simulink model "helicopter_EKF"  (R2021b)
settings: Solver=ode45  StartTime=0.0  StopTime=T  RelTol=1e-3
InitFcn:
  | hwinit
values from neighbouring files (symbols this model uses):
  C = [1, 0, 0; 0, 0, 1]    [controller_LQR.m]    (also in controller_check_EKF.m; polish_MPC.m)
  h = 0.01    [controller_LQR.m]    (also in controller_check_EKF.m; observer_check_EKF.m; polish_MPC.m; validation.m)
  K = place(A_lin, B_lin, p_new)    [controller_check_EKF.m]
  u_start = alpha_to_u(alpha_ref)    [controller_LQR.m]
  x_ref = [alpha_ref; alpha_dot_ref; omega_ref]/0.9    [controller_LQR.m]    (also in controller_check_EKF.m = [alpha_ref; alpha_dot_ref; omega_ref]; polish_MPC.m = [alpha_ref; alpha_dot_ref ; omega_ref])
undefined symbols (not defined in the file or in its folder): A_lin, adingain, adinoffs, B_lin, HeliMexHandle
libraries: simulink x1, sharedTrackingLibrary x1, eeGeneralControl x1, dspstat3 x1
settings Model: Creator=fkzhang  LastModifiedBy=lcaric
settings SolverCC: AlgebraicLoopSolver=TrustRegion
settings DataIOCC: LimitDataPoints=on  SaveFormat=Array  ReturnWorkspaceOutputs=off
settings OptimizationCC: BlockReduction=off  BooleanDataType=off  LifeSpan=inf
settings DebuggingCC: SaveWithParameterizedLinksMsg=none  UnderspecifiedInitializationDetection=Classic  MergeDetectMultiDrivingBlocksExec=none  SignalResolutionControl=TryResolveAllWithWarning  AllowSymbolicDim=off  SFUnexpectedBacktrackingDiag=warning  SFNoUnconditionalDefaultTransitionDiag=warning  SFExecutionAtInitializationDiag=none  SFMachineParentedDataDiag=warning  ArithmeticOperatorsInVariantConditions=warning
settings HardwareCC: ProdBitPerPointer=32  ProdBitPerSizeT=32  ProdBitPerPtrDiffT=32  ProdLargestAtomicFloat=None  ProdIntDivRoundTo=Undefined  ProdEndianess=Unspecified  ProdWordSize=32  ProdHWDeviceType=32-bit Generic  TargetUnknown=on
settings ModelReferenceCC: PropagateSignalLabelsOutOfModel=off
settings SFSimCC: SimUseLocalCustomCode=off  CustomCodeUndefinedFunction=UseInterfaceOnly
settings RTWCC: RTWUseLocalCustomCode=off
settings CodeAppCC: StateflowObjectComments=on
settings GRTTargetCC: TargetLangStandard=C89/C90 (ANSI)
settings ConfigComp: CovMetricSettings=dw  CovSaveCumulativeToWorkspaceVar=on  CovSaveSingleToWorkspaceVar=on  CovExternalEMLEnable=off  CovSFcnEnable=off

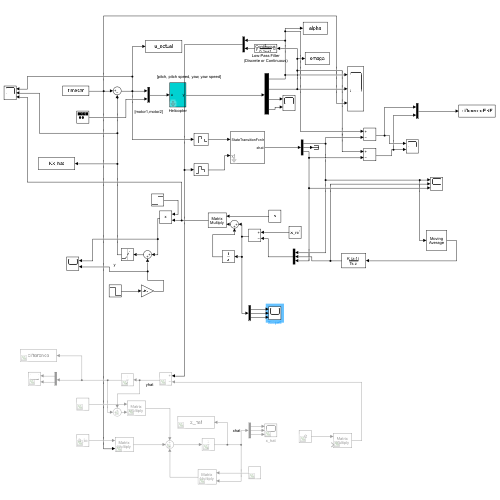
[thumbnail: Simulink's stored preview of the top-level diagram]
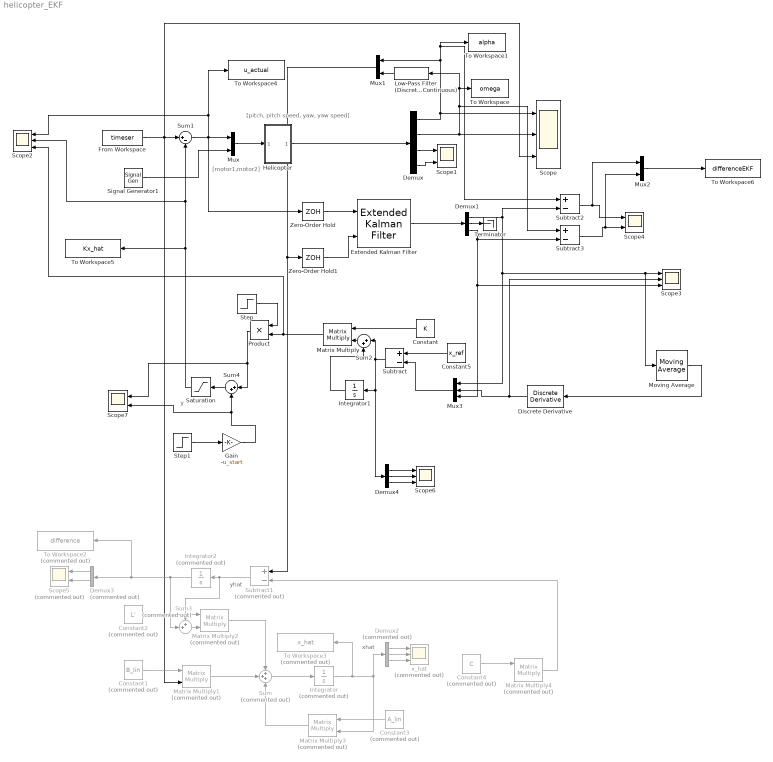
== system helicopter_EKF ==
  note: yhat
  note: y
  note: xhat
  note: [pitch, pitch speed, yaw, yaw speed]
  note: [motor1,motor2]
  Constant : Constant  Value=K  VectorParams1D=off
  Constant1 : Constant  Commented=on  Value=B_lin  VectorParams1D=off
  Constant2 : Constant  Commented=on  Value=L'
  Constant3 : Constant  Commented=on  Value=A_lin
  Constant4 : Constant  Commented=on  Value=C
  Constant5 : Constant  Value=x_ref
  Demux : Demux
  Demux1 : Demux  Outputs=3
  Demux2 : Demux  Commented=on  Outputs=3
  Demux3 : Demux  Commented=on  Outputs=2
  Demux4 : Demux  Outputs=3
  Discrete Derivative : simulink/Discrete/Discrete Derivative  gainval=1.0  ICPrevScaledInput=0.0  OutMin=[]  OutMax=[]  OutDataType=fixdt(1, 16)  OutScaling=2^-10  DoSatur=off
  Extended Kalman Filter : sharedTrackingLibrary/Extended Kalman Filter  StateTransitionFcn=nonlin_evolution  HasStateTransitionJacobianFcn=off  StateTransitionJacobianFcn=nonlin_jacobian  HasAdditiveProcessNoise=Additive  ProcessNoise=Q  HasTimeVaryingProcessNoise=off  HasStateTransitionFcnExtraArgument=1  InitialState=[0; 0; 0]  InitialStateCovariance=Q  MeasurementFcn1=nonlin_measurement_all  HasMeasurementJacobianFcn1=off  HasMeasurementEnablePort1=off  HasAdditiveMeasurementNoise1=Additive  MeasurementNoise1=R  HasTimeVaryingMeasurementNoise1=off  HasMeasurementFcnExtraArgument1=0  MeasurementFcn2=nonlin_measurement_omega  HasMeasurementJacobianFcn2=off  HasMeasurementEnablePort2=off  HasAdditiveMeasurementNoise2=Additive  MeasurementNoise2=10  HasTimeVaryingMeasurementNoise2=off  HasMeasurementFcnExtraArgument2=0  MeasurementFcn3=myMeasurementFcn  HasMeasurementJacobianFcn3=off  HasMeasurementEnablePort3=off  HasAdditiveMeasurementNoise3=Additive  MeasurementNoise3=1  HasTimeVaryingMeasurementNoise3=off  HasMeasurementFcnExtraArgument3=0  MeasurementFcn4=myMeasurementFcn  HasMeasurementJacobianFcn4=off  HasMeasurementEnablePort4=off  HasAdditiveMeasurementNoise4=Additive  MeasurementNoise4=1  HasTimeVaryingMeasurementNoise4=off  HasMeasurementFcnExtraArgument4=0  MeasurementFcn5=myMeasurementFcn  HasMeasurementJacobianFcn5=off  HasMeasurementEnablePort5=off  HasAdditiveMeasurementNoise5=Additive  MeasurementNoise5=1  HasTimeVaryingMeasurementNoise5=off  HasMeasurementFcnExtraArgument5=0  EnableMultirate=off  StateTransitionFcnSampleTime=1  MeasurementFcn1SampleTime=1  MeasurementFcn2SampleTime=1  MeasurementFcn3SampleTime=1  MeasurementFcn4SampleTime=1  MeasurementFcn5SampleTime=1  UseCurrentEstimator=on  OutputStateCovariance=off  DataType=double  SampleTime=0.02  NumberOfMeasurements=1
      settings: SourceProductBaseCode=AE,PW,CT,DR,TF,ID,LP,NV,AR,RO,RR,UV,VE
  From Workspace : FromWorkspace  VariableName=timeser
  Gain : Gain  Gain=-u_start
  Helicopter : Subsystem  mask{Ts=h}
      mask prompts: Ts "sampletime"
      mask init:
      | sf_heli_init
      mask Display:
      | port_label('input',1,'u');
      | port_label('output',1,'y');
  Integrator : Integrator  Commented=on
  Integrator1 : Integrator
  Integrator2 : Integrator  Commented=on
  Low-Pass Filter (Discrete or Continuous) : eeGeneralControl/Low-Pass Filter (Discrete or Continuous)  K=1  T=0.1  B=inf  A=-inf  init_option=Inherited from block input  x0=0  Ts=0
  Matrix Multiply : Product  Multiplication=Matrix(*)
  Matrix Multiply{1..4} (4 alike) : Product  Commented=on  Multiplication=Matrix(*)
  Moving Average : dspstat3/Moving Average  Method=Sliding window  ForgettingFactorPort=off  SpecifyWindowLength=on  WindowLength=5  ForgettingFactor=0.9  SimulateUsing=Code generation
  Mux : Mux  Inputs=2
  Mux1 : Mux  Inputs=2
  Mux2 : Mux  Inputs=2
  Mux3 : Mux  Inputs=3
  Product : Product
  Saturation : Saturate  UpperLimit=1  LowerLimit=-1
  Scope{,2..3,6} (4 alike) : Scope  NumInputPorts=3
  Scope1 : Scope  NumInputPorts=2
  Scope4 : Scope  NumInputPorts=2
  Scope5 : Scope  Commented=on  NumInputPorts=2
  Scope7 : Scope  NumInputPorts=2
  Signal Generator1 : SignalGenerator  WaveForm=square  Amplitude=0  Frequency=1/20
  Step : Step  SampleTime=0
  Step1 : Step  Before=1  After=0  SampleTime=0
  Subtract : Sum  Inputs=+-
  Subtract1 : Sum  Commented=on  Inputs=+-
  Subtract2 : Sum  Inputs=+-
  Subtract3 : Sum  Inputs=+-
  Sum : Sum  Commented=on  Inputs=+++
  Sum1 : Sum  Inputs=|+-
  Sum2 : Sum  Inputs=|++
  Sum3 : Sum  Commented=on  Inputs=++|
  Sum4 : Sum  Inputs=|++
  Terminator : Terminator
  To Workspace : ToWorkspace  VariableName=omega  SaveFormat=Timeseries  SampleTime=-1
  To Workspace1 : ToWorkspace  VariableName=alpha  SaveFormat=Timeseries  SampleTime=-1
  To Workspace2 : ToWorkspace  Commented=on  VariableName=difference  SaveFormat=Timeseries  SampleTime=-1
  To Workspace3 : ToWorkspace  Commented=on  VariableName=x_hat  SaveFormat=Timeseries  SampleTime=-1
  To Workspace4 : ToWorkspace  VariableName=u_actual  SaveFormat=Timeseries  SampleTime=-1
  To Workspace5 : ToWorkspace  VariableName=Kx_hat  SaveFormat=Timeseries  SampleTime=-1
  To Workspace6 : ToWorkspace  VariableName=differenceEKF  SaveFormat=Timeseries  SampleTime=-1
  Zero-Order Hold : ZeroOrderHold  SampleTime=0.02
  Zero-Order Hold1 : ZeroOrderHold  SampleTime=0.02
  x_hat : Scope  Commented=on  NumInputPorts=3
  wires:
  Mux/1 -> Helicopter/1(In1)
  Signal Generator1/1 -> Mux/2
  Demux/2 -> Low-Pass Filter (Discrete or Continuous)/1, To Workspace/1, Subtract3/1, Scope/2
  Demux/3 -> Scope1/1
  Demux/4 -> Scope1/2
  From Workspace/1 -> Sum1/1, Matrix Multiply1/2, Scope/3
  Demux/1 -> Subtract2/1, To Workspace1/1, Mux1/1, Scope/1
  Mux1/1 -> Subtract1/1, Zero-Order Hold1/1
  Helicopter/1(Out1) -> Demux/1
  Matrix Multiply1/1 -> Sum/2
  Matrix Multiply2/1 -> Sum/1
  Sum/1 -> Integrator/1
  Matrix Multiply3/1 -> Sum/3
  Integrator/1 -> To Workspace3/1, Matrix Multiply3/2, Demux2/1
  Demux2/2 -> x_hat/2
  Demux2/3 -> x_hat/3
  Demux2/1 -> x_hat/1
  Subtract1/1 -> Sum3/1, Integrator2/1
  Matrix Multiply4/1 -> Subtract1/2
  Demux3/2 -> Scope5/2
  Demux3/1 -> Scope5/1
  Constant1/1 -> Matrix Multiply1/1
  Constant2/1 -> Matrix Multiply2/1
  Constant4/1 -> Matrix Multiply4/1
  Constant3/1 -> Matrix Multiply3/1
  Sum1/1 -> To Workspace4/1, Scope2/1, Zero-Order Hold/1, Mux/1
  Constant/1 -> Matrix Multiply/1
  Saturation/1 -> To Workspace5/1, Scope2/2, Sum1/2
  Constant5/1 -> Subtract/1
  Sum2/1 -> Matrix Multiply/2
  Integrator2/1 -> Sum3/2, To Workspace2/1, Demux3/1
  Sum3/1 -> Matrix Multiply2/2
  Zero-Order Hold/1 -> Extended Kalman Filter/1
  Zero-Order Hold1/1 -> Extended Kalman Filter/2
  Extended Kalman Filter/1 -> Demux1/1
  Demux1/3 -> Subtract3/2, Mux3/3, Scope3/3
  Subtract2/1 -> Mux2/1, Scope4/1
  Subtract3/1 -> Mux2/2, Scope4/2
  Mux2/1 -> To Workspace6/1
  Low-Pass Filter (Discrete or Continuous)/1 -> Mux1/2
  Demux1/1 -> Subtract2/2, Mux3/1, Moving Average/1, Scope3/1
  Discrete Derivative/1 -> Scope3/2, Mux3/2
  Mux3/1 -> Subtract/2
  Moving Average/1 -> Discrete Derivative/1
  Step/1 -> Product/1
  Product/1 -> Scope7/1, Sum4/1
  Sum4/1 -> Saturation/1
  Step1/1 -> Gain/1
  Gain/1 -> Scope7/2, Sum4/2
  Demux1/2 -> Terminator/1
  Demux4/1 -> Scope6/1
  Demux4/3 -> Scope6/3
  Demux4/2 -> Scope6/2
  Subtract/1 -> Integrator1/1, Demux4/1, Sum2/1
  Integrator1/1 -> Sum2/2
  Matrix Multiply/1 -> Scope2/3, Product/2

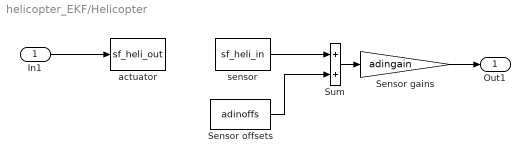
== system helicopter_EKF/Helicopter ==
  In1 : Inport
  Sensor gains : Gain  Gain=adingain
  Sensor offsets : Constant  Value=adinoffs
  Sum : Sum
  actuator : M-S-Function  FunctionName=sf_heli_out  Parameters=HeliMexHandle,Ts
  sensor : M-S-Function  FunctionName=sf_heli_in  Parameters=HeliMexHandle
  Out1 : Outport  VectorParamsAs1DForOutWhenUnconnected=off
  wires:
  sensor/1 -> Sum/1
  In1/1 -> actuator/1
  Sensor offsets/1 -> Sum/2
  Sum/1 -> Sensor gains/1
  Sensor gains/1 -> Out1/1
